simulink model "hydroRotSoln"  (R2015a)
settings: Solver=ode23t  StartTime=0.0  StopTime=100  RelTol=1e-3  AbsTol=1e-3
libraries: fl_lib x12, nesl_utility x3
settings Model: CovSFcnEnable=off  Creator=jrivitus  LastModifiedBy=sseshadr
settings OptimizationCC: ExpressionDepthLimit=2147483647
settings DebuggingCC: UnderspecifiedInitializationDetection=Classic  MergeDetectMultiDrivingBlocksExec=none  ParameterPrecisionLossMsg=none  FcnCallInpInsideContextMsg=UseLocalSettings  StateNameClashWarn=warning
settings GRTTargetCC: CombineOutputUpdateFcns=off  GRTInterface=on

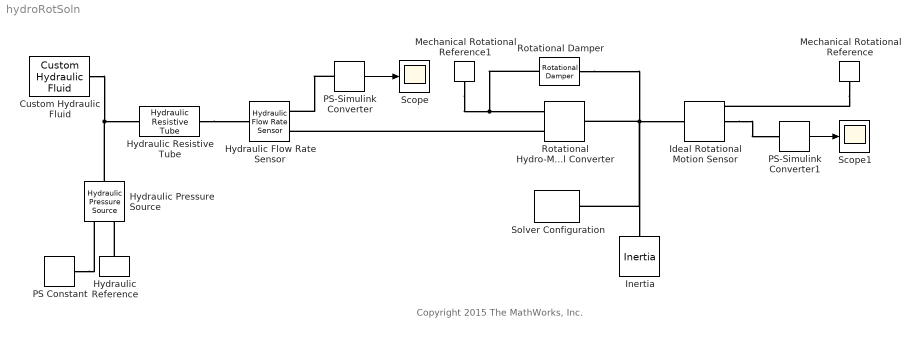
== system hydroRotSoln ==
  note: Copyright 2015 The MathWorks, Inc.
  Custom Hydraulic Fluid : fl_lib/Hydraulic/Hydraulic Utilities/Custom Hydraulic Fluid  density=997 kg/m^3  viscosity_kin=1e-6 m^2/s  bulk=2.2e9 Pa  alpha=0.005  range_error=2
  Hydraulic Flow Rate Sensor : fl_lib/Hydraulic/Hydraulic Sensors/Hydraulic Flow Rate Sensor
  Hydraulic Pressure Source : fl_lib/Hydraulic/Hydraulic Sources/Hydraulic Pressure Source
  Hydraulic Reference : fl_lib/Hydraulic/Hydraulic Elements/Hydraulic Reference
  Hydraulic Resistive Tube : fl_lib/Hydraulic/Hydraulic Elements/Hydraulic Resistive Tube  cs_type=1  d_in=0.1 m  area=1e-4 m^2  D_h=0.0112 m  s_factor=64  length=5 m  length_ad=1 m  roughness=1.5e-5 m  Re_lam=2e+3  Re_turb=4e+3  length_eff=6 m  rel_roughness=0.001  q_specify=off  q_priority=High  q=1e-3 m^3/s  p_specify=off  p_priority=High  p=0 Pa
  Ideal Rotational Motion Sensor : fl_lib/Mechanical/Mechanical Sensors/Ideal Rotational Motion Sensor  offset=0 rad
  Inertia : fl_lib/Mechanical/Rotational Elements/Inertia  inertia=0.01 kg*m^2  w_specify=on  w_priority=High  w=0 rad/s  t_specify=off  t_priority=High  t=0 N*m
  Mechanical Rotational Reference : fl_lib/Mechanical/Rotational Elements/Mechanical Rotational Reference
  Mechanical Rotational Reference1 : fl_lib/Mechanical/Rotational Elements/Mechanical Rotational Reference
  PS Constant : fl_lib/Physical Signals/Sources/PS Constant  constant=100
  PS-Simulink Converter : nesl_utility/PS-Simulink Converter  PhysicalDomain=network_engine_domain  SubClassName=ps_output  LeftPortType=input  RightPortType=output  PseudoPeriodic=off  Frequencies=[]  Unit=m^3/s  AffineConversion=off
  PS-Simulink Converter1 : nesl_utility/PS-Simulink Converter  PhysicalDomain=network_engine_domain  SubClassName=ps_output  LeftPortType=input  RightPortType=output  PseudoPeriodic=off  Frequencies=[]  Unit=rad/s  AffineConversion=off
  Rotational Hydro-Mechanical Converter : fl_lib/Hydraulic/Hydraulic Elements/Rotational Hydro-Mechanical Converter  D=0.0003 m^3/rad  or=1  compressibility=0  initial_angle=0 rad  V_dead=1e-4 m^3  k_sh=1.4  initial_pressure=0 Pa
  Rotational Damper : fl_lib/Mechanical/Rotational Elements/Rotational Damper  D=0.001 N*m/(rad/s)  w_specify=off  w_priority=High  w=0 rad/s  t_specify=off  t_priority=High  t=0 N*m
  Scope : Scope
      settings: TimeRange=100  YMin=0  YMax=0.003
  Scope1 : Scope
      settings: TimeRange=100  YMin=0  YMax=10
  Solver Configuration : nesl_utility/Solver Configuration  PhysicalDomain=network_engine_domain  SubClassName=solver  LeftPortType=input  RightPortType=generic  Accelerate=off  Tones=[]  Harmonics=[]  SimulateNoise=off  Profile=off  UseLocalSampling=off  EnableSwitchedLinearOptims=on  FrequencyDomain=off  UseCCode=off  RelTol=0.001  AbsTol=1e-06  MinStep=1e-09  ToWorkspace=off  RevertToSquareIcSolve=off  NumHomotopyIterations=100  DoDC=off  ResidualTolerance=1e-9  UseLocalSolver=off  LocalSolverChoice=NE_BACKWARD_EULER_ADVANCER  LocalSolverSampleTime=.001  DoFixedCost=off  MaxNonlinIter=3  MaxModeIter=2  LinearAlgebra=Sparse  DelaysMemoryBudget=1024  AutomaticFiltering=on  FilteringTimeConstant=0.001
  wires:
  PS-Simulink Converter/1 -> Scope/1
  PS-Simulink Converter1/1 -> Scope1/1
  connections:
  Hydraulic Pressure Source/LConn1 -- Hydraulic Resistive Tube/LConn1 -- Custom Hydraulic Fluid/RConn1
  PS Constant/RConn1 -- Hydraulic Pressure Source/RConn1
  Hydraulic Resistive Tube/RConn1 -- Hydraulic Flow Rate Sensor/LConn1
  PS-Simulink Converter/LConn1 -- Hydraulic Flow Rate Sensor/RConn1
  Hydraulic Reference/LConn1 -- Hydraulic Pressure Source/RConn2
  Ideal Rotational Motion Sensor/RConn2 -- PS-Simulink Converter1/LConn1
  Mechanical Rotational Reference/LConn1 -- Ideal Rotational Motion Sensor/RConn1
  Rotational Damper/LConn1 -- Rotational Hydro-Mechanical Converter/RConn1 -- Solver Configuration/RConn1 -- Inertia/LConn1 -- Ideal Rotational Motion Sensor/LConn1
  Mechanical Rotational Reference1/LConn1 -- Rotational Damper/RConn1 -- Rotational Hydro-Mechanical Converter/LConn1
  Rotational Hydro-Mechanical Converter/LConn2 -- Hydraulic Flow Rate Sensor/RConn2
